simulink model "Zad1"  (R2020b)
settings: Solver=VariableStepAuto  StartTime=0.0  StopTime=0.0  RelTol=1e-3
libraries: CPOiS_SourcesSinks x11, CPOiS_DataManipulation_DataTypeConversion x7, CPOiS_LinearTransforms x6, CPOiS_DataManipulation_IntroduceNoise x2, CPOiS_General x1
settings Model: Creator=Krystian  LastModifiedBy=Krystian

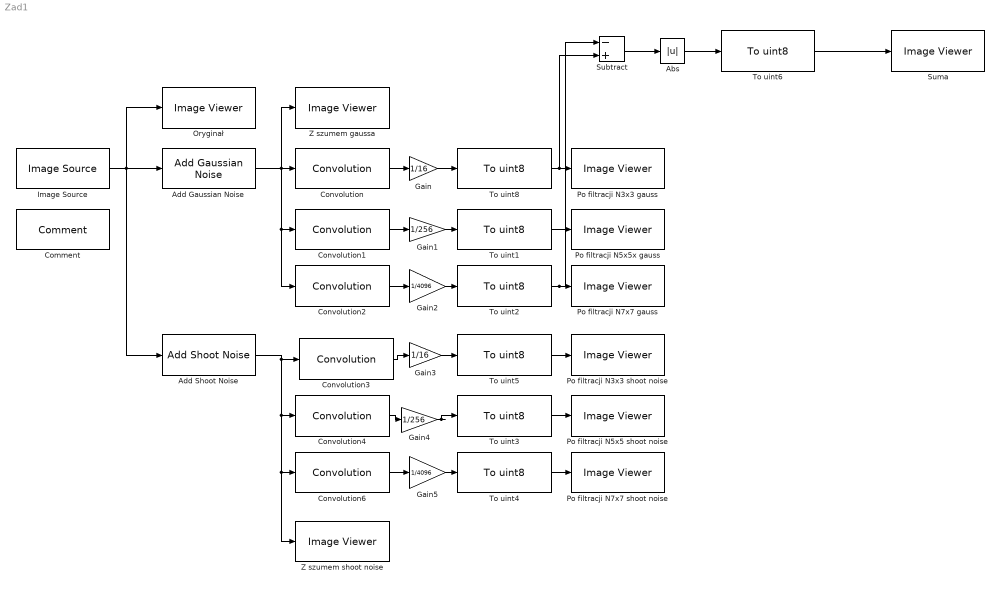
== system Zad1 ==
  Abs : Abs
  Add Gaussian Noise : CPOiS_DataManipulation_IntroduceNoise/Add Gaussian Noise  Mean=0  Variance=1
      settings: SourceProductName=CPOiS - Digital image and signal processing
  Add Shoot Noise : CPOiS_DataManipulation_IntroduceNoise/Add Shoot Noise  Density=5
      settings: SourceProductName=CPOiS - Digital image and signal processing
  Comment : CPOiS_General/Comment
      settings: SourceProductName=CPOiS - Digital image and signal processing
  Convolution : CPOiS_LinearTransforms/Convolution  ConvolutionMatrix=[1,2,1;2,4,2;1,2,1]
      settings: SourceProductName=CPOiS - Digital image and signal processing
  Convolution1 : CPOiS_LinearTransforms/Convolution  ConvolutionMatrix=[1,4,6,4,1;4,16,24,16,4;6,24,36,24,6;4,16,24,16,4;1,4,6,4,1]
      settings: SourceProductName=CPOiS - Digital image and signal processing
  Convolution2 : CPOiS_LinearTransforms/Convolution  ConvolutionMatrix=[1,6,15,20,15,6,1;6,36,90,120,90,36,6;15,90,225,300,225,90,15;20,120,300,400,300,120,20;15,90,225,300,225,90,15;6,36,90,120,90,36,6;1,6,15,20,15,6,1]
      settings: SourceProductName=CPOiS - Digital image and signal processing
  Convolution3 : CPOiS_LinearTransforms/Convolution  ConvolutionMatrix=[1,2,1;2,4,2;1,2,1]
      settings: SourceProductName=CPOiS - Digital image and signal processing
  Convolution4 : CPOiS_LinearTransforms/Convolution  ConvolutionMatrix=[1,4,6,4,1;4,16,24,16,4;6,24,36,24,6;4,16,24,16,4;1,4,6,4,1]
      settings: SourceProductName=CPOiS - Digital image and signal processing
  Convolution6 : CPOiS_LinearTransforms/Convolution  ConvolutionMatrix=[1,6,15,20,15,6,1;6,36,90,120,90,36,6;15,90,225,300,225,90,15;20,120,300,400,300,120,20;15,90,225,300,225,90,15;6,36,90,120,90,36,6;1,6,15,20,15,6,1]
      settings: SourceProductName=CPOiS - Digital image and signal processing
  Gain : Gain  Gain=1/16
  Gain1 : Gain  Gain=1/256
  Gain2 : Gain  Gain=1/4096  OutDataTypeStr=double  RndMeth=Nearest
  Gain3 : Gain  Gain=1/16
  Gain4 : Gain  Gain=1/256
  Gain5 : Gain  Gain=1/4096  OutDataTypeStr=double  RndMeth=Nearest
  Image Source : CPOiS_SourcesSinks/Image Source  FileSelection=ball.png
      settings: SourceProductName=CPOiS - Digital image and signal processing
  Oryginał : CPOiS_SourcesSinks/Image Viewer
      settings: SourceProductName=CPOiS - Digital image and signal processing
  Po filtracji N3x3 gauss : CPOiS_SourcesSinks/Image Viewer
      settings: SourceProductName=CPOiS - Digital image and signal processing
  Po filtracji N3x3 shoot noise : CPOiS_SourcesSinks/Image Viewer
      settings: SourceProductName=CPOiS - Digital image and signal processing
  Po filtracji N5x5 shoot noise : CPOiS_SourcesSinks/Image Viewer
      settings: SourceProductName=CPOiS - Digital image and signal processing
  Po filtracji N5x5x gauss : CPOiS_SourcesSinks/Image Viewer
      settings: SourceProductName=CPOiS - Digital image and signal processing
  Po filtracji N7x7 gauss : CPOiS_SourcesSinks/Image Viewer
      settings: SourceProductName=CPOiS - Digital image and signal processing
  Po filtracji N7x7 shoot noise : CPOiS_SourcesSinks/Image Viewer
      settings: SourceProductName=CPOiS - Digital image and signal processing
  Subtract : Sum  Inputs=-+
  Suma : CPOiS_SourcesSinks/Image Viewer
      settings: SourceProductName=CPOiS - Digital image and signal processing
  To uint{1..6,8} (7 alike) : CPOiS_DataManipulation_DataTypeConversion/To uint8
      settings: SourceProductName=CPOiS - Digital image and signal processing
  "Z szumem gaussa " : CPOiS_SourcesSinks/Image Viewer
      settings: SourceProductName=CPOiS - Digital image and signal processing
  Z szumem shoot noise : CPOiS_SourcesSinks/Image Viewer
      settings: SourceProductName=CPOiS - Digital image and signal processing
  wires:
  To uint3/1 -> Po filtracji N5x5 shoot noise/1
  Convolution3/1 -> Gain3/1
  Convolution6/1 -> Gain5/1
  To uint2/1 -> Subtract/1, Po filtracji N7x7 gauss/1
  To uint5/1 -> Po filtracji N3x3 shoot noise/1
  To uint1/1 -> Po filtracji N5x5x gauss/1
  Add Gaussian Noise/1 -> Convolution1/1, Convolution2/1, Convolution/1, "Z szumem gaussa "/1
  Add Shoot Noise/1 -> Convolution3/1, Convolution4/1, Z szumem shoot noise/1, Convolution6/1
  Gain2/1 -> To uint2/1
  Convolution1/1 -> Gain1/1
  Convolution/1 -> Gain/1
  Convolution2/1 -> Gain2/1
  Gain5/1 -> To uint4/1
  Gain1/1 -> To uint1/1
  Gain/1 -> To uint8/1
  Image Source/1 -> Add Shoot Noise/1, Add Gaussian Noise/1, Oryginał/1
  Gain3/1 -> To uint5/1
  To uint4/1 -> Po filtracji N7x7 shoot noise/1
  Gain4/1 -> To uint3/1
  Convolution4/1 -> Gain4/1
  To uint6/1 -> Suma/1
  Subtract/1 -> Abs/1
  Abs/1 -> To uint6/1
  To uint8/1 -> Subtract/2, Po filtracji N3x3 gauss/1
